simulink subsystem "VCM_main"  (R2021b)
settings: Solver=VariableStepAuto  StartTime=0.0  StopTime=10.0  RelTol=1e-3
undefined symbols (not defined in the file): df, dr, g, gear_f, gear_r, Iwf, Iwr, l, lf, M, Rwf, Rwr
libraries: simulink x47, dspstat3 x2, dspswit3 x1
(part 2 of 4)

== system VCM_main/Sequence/bInberterOn_SwBox1 ==
  BUS : Inport
  error sig1 : Inport  Port=2
  error sig2 : Inport  Port=3
  error sig3 : Inport  Port=4
  error sig4 : Inport  Port=5
  Bus Selector2 : BusSelector  OutputSignals=MC1_sw,MC2_sw,MC3_sw,MC4_sw
  Constant : Constant
  Switch{1..4} (4 alike) : Switch  Criteria=u2 > Threshold
  Out1 : Outport  VectorParamsAs1DForOutWhenUnconnected=off
  Out2 : Outport  Port=2  VectorParamsAs1DForOutWhenUnconnected=off
  Out3 : Outport  Port=3  VectorParamsAs1DForOutWhenUnconnected=off
  Out4 : Outport  Port=4  VectorParamsAs1DForOutWhenUnconnected=off
  wires:
  error sig2/1 -> Switch2/1
  error sig3/1 -> Switch3/1
  error sig4/1 -> Switch4/1
  BUS/1 -> Bus Selector2/1
  Bus Selector2/4 -> Switch4/2  "<MC4_sw>"
  Bus Selector2/3 -> Switch3/2  "<MC3_sw>"
  Bus Selector2/1 -> Switch1/2  "<MC1_sw>"
  Bus Selector2/2 -> Switch2/2  "<MC2_sw>"
  Switch3/1 -> Out3/1
  Switch2/1 -> Out2/1
  error sig1/1 -> Switch1/1
  Switch1/1 -> Out1/1
  Switch4/1 -> Out4/1
  Constant/1 -> Switch1/3, Switch2/3, Switch3/3, Switch4/3

== system VCM_main/Sequence/bQuitDcOn_SwBox ==
  BUS : Inport
  error sig1 : Inport  Port=2
  error sig2 : Inport  Port=3
  error sig3 : Inport  Port=4
  error sig4 : Inport  Port=5
  Bus Selector2 : BusSelector  OutputSignals=MC1_sw,MC2_sw,MC3_sw,MC4_sw
  Constant : Constant
  Switch{1..4} (4 alike) : Switch  Criteria=u2 > Threshold
  Out1 : Outport  VectorParamsAs1DForOutWhenUnconnected=off
  Out2 : Outport  Port=2  VectorParamsAs1DForOutWhenUnconnected=off
  Out3 : Outport  Port=3  VectorParamsAs1DForOutWhenUnconnected=off
  Out4 : Outport  Port=4  VectorParamsAs1DForOutWhenUnconnected=off
  wires:
  error sig2/1 -> Switch2/1
  error sig3/1 -> Switch3/1
  error sig4/1 -> Switch4/1
  BUS/1 -> Bus Selector2/1
  Bus Selector2/4 -> Switch4/2  "<MC4_sw>"
  Bus Selector2/3 -> Switch3/2  "<MC3_sw>"
  Bus Selector2/1 -> Switch1/2  "<MC1_sw>"
  Bus Selector2/2 -> Switch2/2  "<MC2_sw>"
  Switch3/1 -> Out3/1
  Switch2/1 -> Out2/1
  error sig1/1 -> Switch1/1
  Switch1/1 -> Out1/1
  Switch4/1 -> Out4/1
  Constant/1 -> Switch1/3, Switch2/3, Switch3/3, Switch4/3

== system VCM_main/Sequence/bSystemReady_SwBox ==
  BUS : Inport
  error sig1 : Inport  Port=2
  error sig2 : Inport  Port=3
  error sig3 : Inport  Port=4
  error sig4 : Inport  Port=5
  Bus Selector2 : BusSelector  OutputSignals=MC1_sw,MC2_sw,MC3_sw,MC4_sw
  Constant : Constant
  Switch{1..4} (4 alike) : Switch  Criteria=u2 > Threshold
  Out1 : Outport  VectorParamsAs1DForOutWhenUnconnected=off
  Out2 : Outport  Port=2  VectorParamsAs1DForOutWhenUnconnected=off
  Out3 : Outport  Port=3  VectorParamsAs1DForOutWhenUnconnected=off
  Out4 : Outport  Port=4  VectorParamsAs1DForOutWhenUnconnected=off
  wires:
  error sig2/1 -> Switch2/1
  error sig3/1 -> Switch3/1
  error sig4/1 -> Switch4/1
  BUS/1 -> Bus Selector2/1
  Bus Selector2/4 -> Switch4/2  "<MC4_sw>"
  Bus Selector2/3 -> Switch3/2  "<MC3_sw>"
  Bus Selector2/1 -> Switch1/2  "<MC1_sw>"
  Bus Selector2/2 -> Switch2/2  "<MC2_sw>"
  Switch3/1 -> Out3/1
  Switch2/1 -> Out2/1
  error sig1/1 -> Switch1/1
  Switch1/1 -> Out1/1
  Switch4/1 -> Out4/1
  Constant/1 -> Switch1/3, Switch2/3, Switch3/3, Switch4/3

== system VCM_main/Speed Torque MC1/Power limit Negative ==
  Speed : Inport
  Trq : Inport  Port=2
  Constant : Constant  Value=-10000
  Fcn : Fcn  Expr=u(1)/(2*pi*u(2)/60)
  Saturation : Saturate  UpperLimit=30000  LowerLimit=1
  Saturation Dynamic : simulink/Discontinuities/Saturation Dynamic  OutMin=[]  OutMax=[]  OutDataTypeStr=Inherit: Same as second input  OutDataType=fixdt(1, 16)  OutScaling=2^-10  DoSatur=off
  Vector Concatenate : Concatenate
  power limit : Constant  Value=0
  Out1 : Outport  VectorParamsAs1DForOutWhenUnconnected=off
  wires:
  Saturation/1 -> Vector Concatenate/2
  Fcn/1 -> Saturation Dynamic/3
  Vector Concatenate/1 -> Fcn/1
  Constant/1 -> Vector Concatenate/1
  Speed/1 -> Saturation/1
  Saturation Dynamic/1 -> Out1/1
  power limit/1 -> Saturation Dynamic/1
  Trq/1 -> Saturation Dynamic/2

== system VCM_main/Speed Torque MC1/Power limit Positive ==
  note: 80kWPowerLimitがoffのとき
      | モーター1つあたりの出力＊効率
  note: 80kWPowerLimitがonのとき
      | モーター単体最高出力＊効率
  note: PositiveTrqLimitは
      | 単体出力を超えない
      | かつ0以上
  note: 0割り防ぐためだけ
  Trq : Inport
  Speed : Inport  Port=2
  Constant1 : Constant  Value=0
  Fcn : Fcn  Expr=u(1)/(2*pi*u(2)/60)
  Saturation : Saturate  UpperLimit=30000  LowerLimit=1
  Saturation Dynamic : simulink/Discontinuities/Saturation Dynamic  OutMin=[]  OutMax=[]  OutDataTypeStr=Inherit: Same as second input  OutDataType=fixdt(1, 16)  OutScaling=2^-10  DoSatur=off
  Switch : Switch  Criteria=u2 > Threshold  Threshold=0.5
  Vector Concatenate : Concatenate
  all power limit : Constant  Value=35000*0.6
  "each power limit " : Constant  Value=80000/4*0.7
  Out1 : Outport  VectorParamsAs1DForOutWhenUnconnected=off
  wires:
  all power limit/1 -> Switch/1
  "each power limit "/1 -> Switch/3
  [PowerLimitOn] -> Switch/2
  Saturation/1 -> Vector Concatenate/2
  Trq/1 -> Saturation Dynamic/2
  Vector Concatenate/1 -> Fcn/1
  Fcn/1 -> Saturation Dynamic/1
  Switch/1 -> Vector Concatenate/1
  Speed/1 -> Saturation/1
  Saturation Dynamic/1 -> Out1/1
  Constant1/1 -> Saturation Dynamic/3

== system VCM_main/Speed Torque MC1/Subsystem ==
  note: 整数にするときに四捨五入してしまったので
      | インバーターに送って良い最大トルク指令値(0.1%Mn)の2142を
      | 超えることがあるのでminを入れた。
      | 2142より大きい値を送るとエラー出る。
  Positive torque limit : Inport
  M set point MAX 0.1%Mn : Constant  Value=2142
  MinMax : MinMax  Inputs=2
  Positive torque limit1 : Outport  VectorParamsAs1DForOutWhenUnconnected=off
  wires:
  MinMax/1 -> Positive torque limit1/1  "Positive torque limit"
  Positive torque limit/1 -> MinMax/1
  M set point MAX 0.1%Mn/1 -> MinMax/2

== system VCM_main/Speed Torque MC1/TargetVelocity ==
  note: なぜあるかわからん
      | byそが
  note: トルク指令値が正なら
      | SpeedSetpointはTargetSpeedに
      | トルク指令値が負なら
      | SpeedSetpointは0に
  trq : Inport
  target speed : Inport  Port=2
  Constant1 : Constant  Value=0
  Delay : Delay  DelayLength=1  InitialCondition=0
  MinMax : MinMax  Inputs=2
  Switch : Switch  Criteria=u2 > Threshold
  SpeedSetpoint : Outport  VectorParamsAs1DForOutWhenUnconnected=off
  wires:
  MinMax/1 -> SpeedSetpoint/1
  Delay/1 -> MinMax/2
  Switch/1 -> Delay/1, MinMax/1
  Constant1/1 -> Switch/3
  target speed/1 -> Switch/1
  trq/1 -> Switch/2

== system VCM_main/Speed Torque MC1/Torque delay N ==
  In1 : Inport
  Delay : Delay  DelayLength=1  InitialCondition=0
  MinMax : MinMax  Inputs=2
  Out1 : Outport  VectorParamsAs1DForOutWhenUnconnected=off
  wires:
  MinMax/1 -> Out1/1
  Delay/1 -> MinMax/2
  In1/1 -> Delay/1, MinMax/1

== system VCM_main/Speed Torque MC1/Torque delay P ==
  note: なぜあるかわからん
      | byそが
  In1 : Inport
  Delay : Delay  DelayLength=1  InitialCondition=0
  MinMax : MinMax  Function=max  Inputs=2
  Out1 : Outport  VectorParamsAs1DForOutWhenUnconnected=off
  wires:
  MinMax/1 -> Out1/1
  Delay/1 -> MinMax/2
  In1/1 -> Delay/1, MinMax/1

== system VCM_main/Speed Torque MC2/Power limit Negative ==
  Speed : Inport
  Trq : Inport  Port=2
  Constant : Constant  Value=-10000
  Fcn : Fcn  Expr=u(1)/(2*pi*u(2)/60)
  Saturation : Saturate  UpperLimit=30000  LowerLimit=1
  Saturation Dynamic : simulink/Discontinuities/Saturation Dynamic  OutMin=[]  OutMax=[]  OutDataTypeStr=Inherit: Same as second input  OutDataType=fixdt(1, 16)  OutScaling=2^-10  DoSatur=off
  Vector Concatenate : Concatenate
  power limit : Constant  Value=0
  Out1 : Outport  VectorParamsAs1DForOutWhenUnconnected=off
  wires:
  Trq/1 -> Saturation Dynamic/2
  power limit/1 -> Saturation Dynamic/1
  Saturation Dynamic/1 -> Out1/1
  Speed/1 -> Saturation/1
  Constant/1 -> Vector Concatenate/1
  Vector Concatenate/1 -> Fcn/1
  Fcn/1 -> Saturation Dynamic/3
  Saturation/1 -> Vector Concatenate/2

== system VCM_main/Speed Torque MC2/Power limit Positive ==
  note: 0割り防ぐためだけ
  note: PositiveTrqLimitは
      | 単体出力を超えない
      | かつ0以上
  note: 80kWPowerLimitがonのとき
      | モーター単体最高出力＊効率
  note: 80kWPowerLimitがoffのとき
      | モーター1つあたりの出力＊効率
  Trq : Inport
  Speed : Inport  Port=2
  Constant1 : Constant  Value=0
  Fcn : Fcn  Expr=u(1)/(2*pi*u(2)/60)
  Saturation : Saturate  UpperLimit=30000  LowerLimit=1
  Saturation Dynamic : simulink/Discontinuities/Saturation Dynamic  OutMin=[]  OutMax=[]  OutDataTypeStr=Inherit: Same as second input  OutDataType=fixdt(1, 16)  OutScaling=2^-10  DoSatur=off
  Switch : Switch  Criteria=u2 > Threshold  Threshold=0.5
  Vector Concatenate : Concatenate
  all power limit : Constant  Value=35000*0.6
  "each power limit " : Constant  Value=80000/4*0.7
  Out1 : Outport  VectorParamsAs1DForOutWhenUnconnected=off
  wires:
  Constant1/1 -> Saturation Dynamic/3
  Saturation Dynamic/1 -> Out1/1
  Speed/1 -> Saturation/1
  Switch/1 -> Vector Concatenate/1
  Fcn/1 -> Saturation Dynamic/1
  Vector Concatenate/1 -> Fcn/1
  Trq/1 -> Saturation Dynamic/2
  Saturation/1 -> Vector Concatenate/2
  [PowerLimitOn] -> Switch/2
  "each power limit "/1 -> Switch/3
  all power limit/1 -> Switch/1

== system VCM_main/Speed Torque MC2/Subsystem ==
  note: 整数にするときに四捨五入してしまったので
      | インバーターに送って良い最大トルク指令値(0.1%Mn)の2142を
      | 超えることがあるのでminを入れた。
      | 2142より大きい値を送るとエラー出る。
  Positive torque limit : Inport
  M set point MAX 0.1%Mn : Constant  Value=2142
  MinMax : MinMax  Inputs=2
  Positive torque limit1 : Outport  VectorParamsAs1DForOutWhenUnconnected=off
  wires:
  M set point MAX 0.1%Mn/1 -> MinMax/2
  Positive torque limit/1 -> MinMax/1
  MinMax/1 -> Positive torque limit1/1  "Positive torque limit"

== system VCM_main/Speed Torque MC2/TargetVelocity ==
  note: トルク指令値が正なら
      | SpeedSetpointはTargetSpeedに
      | トルク指令値が負なら
      | SpeedSetpointは0に
  note: なぜあるかわからん
      | byそが
  trq : Inport
  target speed : Inport  Port=2
  Constant1 : Constant  Value=0
  Delay : Delay  DelayLength=1  InitialCondition=0
  MinMax : MinMax  Inputs=2
  Switch : Switch  Criteria=u2 > Threshold
  SpeedSetpoint : Outport  VectorParamsAs1DForOutWhenUnconnected=off
  wires:
  trq/1 -> Switch/2
  target speed/1 -> Switch/1
  Constant1/1 -> Switch/3
  Switch/1 -> MinMax/1, Delay/1
  Delay/1 -> MinMax/2
  MinMax/1 -> SpeedSetpoint/1

== system VCM_main/Speed Torque MC2/Torque delay N ==
  In1 : Inport
  Delay : Delay  DelayLength=1  InitialCondition=0
  MinMax : MinMax  Inputs=2
  Out1 : Outport  VectorParamsAs1DForOutWhenUnconnected=off
  wires:
  In1/1 -> MinMax/1, Delay/1
  Delay/1 -> MinMax/2
  MinMax/1 -> Out1/1

== system VCM_main/Speed Torque MC2/Torque delay P ==
  note: なぜあるかわからん
      | byそが
  In1 : Inport
  Delay : Delay  DelayLength=1  InitialCondition=0
  MinMax : MinMax  Function=max  Inputs=2
  Out1 : Outport  VectorParamsAs1DForOutWhenUnconnected=off
  wires:
  In1/1 -> MinMax/1, Delay/1
  Delay/1 -> MinMax/2
  MinMax/1 -> Out1/1

== system VCM_main/Speed Torque MC3/Power limit Negative ==
  Speed : Inport
  Trq : Inport  Port=2
  Constant : Constant  Value=-10000
  Fcn : Fcn  Expr=u(1)/(2*pi*u(2)/60)
  Saturation : Saturate  UpperLimit=30000  LowerLimit=1
  Saturation Dynamic : simulink/Discontinuities/Saturation Dynamic  OutMin=[]  OutMax=[]  OutDataTypeStr=Inherit: Same as second input  OutDataType=fixdt(1, 16)  OutScaling=2^-10  DoSatur=off
  Vector Concatenate : Concatenate
  power limit : Constant  Value=0
  Out1 : Outport  VectorParamsAs1DForOutWhenUnconnected=off
  wires:
  Saturation/1 -> Vector Concatenate/2
  Fcn/1 -> Saturation Dynamic/3
  Vector Concatenate/1 -> Fcn/1
  Constant/1 -> Vector Concatenate/1
  Speed/1 -> Saturation/1
  Saturation Dynamic/1 -> Out1/1
  power limit/1 -> Saturation Dynamic/1
  Trq/1 -> Saturation Dynamic/2

== system VCM_main/Speed Torque MC3/Power limit Positive ==
  note: 80kWPowerLimitがoffのとき
      | モーター1つあたりの出力＊効率
  note: 80kWPowerLimitがonのとき
      | モーター単体最高出力＊効率
  note: PositiveTrqLimitは
      | 単体出力を超えない
      | かつ0以上
  note: 0割り防ぐためだけ
  Trq : Inport
  Speed : Inport  Port=2
  Constant1 : Constant  Value=0
  Fcn : Fcn  Expr=u(1)/(2*pi*u(2)/60)
  Saturation : Saturate  UpperLimit=30000  LowerLimit=1
  Saturation Dynamic : simulink/Discontinuities/Saturation Dynamic  OutMin=[]  OutMax=[]  OutDataTypeStr=Inherit: Same as second input  OutDataType=fixdt(1, 16)  OutScaling=2^-10  DoSatur=off
  Switch : Switch  Criteria=u2 > Threshold  Threshold=0.5
  Vector Concatenate : Concatenate
  all power limit : Constant  Value=35000*0.6
  "each power limit " : Constant  Value=80000/4*0.7
  Out1 : Outport  VectorParamsAs1DForOutWhenUnconnected=off
  wires:
  all power limit/1 -> Switch/1
  "each power limit "/1 -> Switch/3
  [PowerLimitOn] -> Switch/2
  Saturation/1 -> Vector Concatenate/2
  Trq/1 -> Saturation Dynamic/2
  Vector Concatenate/1 -> Fcn/1
  Fcn/1 -> Saturation Dynamic/1
  Switch/1 -> Vector Concatenate/1
  Speed/1 -> Saturation/1
  Saturation Dynamic/1 -> Out1/1
  Constant1/1 -> Saturation Dynamic/3

== system VCM_main/Speed Torque MC3/Subsystem ==
  note: 整数にするときに四捨五入してしまったので
      | インバーターに送って良い最大トルク指令値(0.1%Mn)の2142を
      | 超えることがあるのでminを入れた。
      | 2142より大きい値を送るとエラー出る。
  Positive torque limit : Inport
  M set point MAX 0.1%Mn : Constant  Value=2142
  MinMax : MinMax  Inputs=2
  Positive torque limit1 : Outport  VectorParamsAs1DForOutWhenUnconnected=off
  wires:
  MinMax/1 -> Positive torque limit1/1  "Positive torque limit"
  Positive torque limit/1 -> MinMax/1
  M set point MAX 0.1%Mn/1 -> MinMax/2

== system VCM_main/Speed Torque MC3/TargetVelocity ==
  note: なぜあるかわからん
      | byそが
  note: トルク指令値が正なら
      | SpeedSetpointはTargetSpeedに
      | トルク指令値が負なら
      | SpeedSetpointは0に
  trq : Inport
  target speed : Inport  Port=2
  Constant1 : Constant  Value=0
  Delay : Delay  DelayLength=1  InitialCondition=0
  MinMax : MinMax  Inputs=2
  Switch : Switch  Criteria=u2 > Threshold
  SpeedSetpoint : Outport  VectorParamsAs1DForOutWhenUnconnected=off
  wires:
  MinMax/1 -> SpeedSetpoint/1
  Delay/1 -> MinMax/2
  Switch/1 -> Delay/1, MinMax/1
  Constant1/1 -> Switch/3
  target speed/1 -> Switch/1
  trq/1 -> Switch/2

== system VCM_main/Speed Torque MC3/Torque delay N ==
  In1 : Inport
  Delay : Delay  DelayLength=1  InitialCondition=0
  MinMax : MinMax  Inputs=2
  Out1 : Outport  VectorParamsAs1DForOutWhenUnconnected=off
  wires:
  MinMax/1 -> Out1/1
  Delay/1 -> MinMax/2
  In1/1 -> Delay/1, MinMax/1

== system VCM_main/Speed Torque MC3/Torque delay P ==
  note: なぜあるかわからん
      | byそが
  In1 : Inport
  Delay : Delay  DelayLength=1  InitialCondition=0
  MinMax : MinMax  Function=max  Inputs=2
  Out1 : Outport  VectorParamsAs1DForOutWhenUnconnected=off
  wires:
  MinMax/1 -> Out1/1
  Delay/1 -> MinMax/2
  In1/1 -> Delay/1, MinMax/1

== system VCM_main/Speed Torque MC4/Power limit Negative ==
  Speed : Inport
  Trq : Inport  Port=2
  Constant : Constant  Value=-10000
  Fcn : Fcn  Expr=u(1)/(2*pi*u(2)/60)
  Saturation : Saturate  UpperLimit=30000  LowerLimit=1
  Saturation Dynamic : simulink/Discontinuities/Saturation Dynamic  OutMin=[]  OutMax=[]  OutDataTypeStr=Inherit: Same as second input  OutDataType=fixdt(1, 16)  OutScaling=2^-10  DoSatur=off
  Vector Concatenate : Concatenate
  power limit : Constant  Value=0
  Out1 : Outport  VectorParamsAs1DForOutWhenUnconnected=off
  wires:
  Trq/1 -> Saturation Dynamic/2
  power limit/1 -> Saturation Dynamic/1
  Saturation Dynamic/1 -> Out1/1
  Speed/1 -> Saturation/1
  Constant/1 -> Vector Concatenate/1
  Vector Concatenate/1 -> Fcn/1
  Fcn/1 -> Saturation Dynamic/3
  Saturation/1 -> Vector Concatenate/2

== system VCM_main/Speed Torque MC4/Power limit Positive ==
  note: 0割り防ぐためだけ
  note: PositiveTrqLimitは
      | 単体出力を超えない
      | かつ0以上
  note: 80kWPowerLimitがonのとき
      | モーター単体最高出力＊効率
  note: 80kWPowerLimitがoffのとき
      | モーター1つあたりの出力＊効率
  Trq : Inport
  Speed : Inport  Port=2
  Constant1 : Constant  Value=0
  Fcn : Fcn  Expr=u(1)/(2*pi*u(2)/60)
  Saturation : Saturate  UpperLimit=30000  LowerLimit=1
  Saturation Dynamic : simulink/Discontinuities/Saturation Dynamic  OutMin=[]  OutMax=[]  OutDataTypeStr=Inherit: Same as second input  OutDataType=fixdt(1, 16)  OutScaling=2^-10  DoSatur=off
  Switch : Switch  Criteria=u2 > Threshold  Threshold=0.5
  Vector Concatenate : Concatenate
  all power limit : Constant  Value=35000*0.6
  "each power limit " : Constant  Value=80000/4*0.7
  Out1 : Outport  VectorParamsAs1DForOutWhenUnconnected=off
  wires:
  Constant1/1 -> Saturation Dynamic/3
  Saturation Dynamic/1 -> Out1/1
  Speed/1 -> Saturation/1
  Switch/1 -> Vector Concatenate/1
  Fcn/1 -> Saturation Dynamic/1
  Vector Concatenate/1 -> Fcn/1
  Trq/1 -> Saturation Dynamic/2
  Saturation/1 -> Vector Concatenate/2
  [PowerLimitOn] -> Switch/2
  "each power limit "/1 -> Switch/3
  all power limit/1 -> Switch/1

== system VCM_main/Speed Torque MC4/Subsystem ==
  note: 整数にするときに四捨五入してしまったので
      | インバーターに送って良い最大トルク指令値(0.1%Mn)の2142を
      | 超えることがあるのでminを入れた。
      | 2142より大きい値を送るとエラー出る。
  Positive torque limit : Inport
  M set point MAX 0.1%Mn : Constant  Value=2142
  MinMax : MinMax  Inputs=2
  Positive torque limit1 : Outport  VectorParamsAs1DForOutWhenUnconnected=off
  wires:
  M set point MAX 0.1%Mn/1 -> MinMax/2
  Positive torque limit/1 -> MinMax/1
  MinMax/1 -> Positive torque limit1/1  "Positive torque limit"

== system VCM_main/Speed Torque MC4/TargetVelocity ==
  note: トルク指令値が正なら
      | SpeedSetpointはTargetSpeedに
      | トルク指令値が負なら
      | SpeedSetpointは0に
  note: なぜあるかわからん
      | byそが
  trq : Inport
  target speed : Inport  Port=2
  Constant1 : Constant  Value=0
  Delay : Delay  DelayLength=1  InitialCondition=0
  MinMax : MinMax  Inputs=2
  Switch : Switch  Criteria=u2 > Threshold
  SpeedSetpoint : Outport  VectorParamsAs1DForOutWhenUnconnected=off
  wires:
  trq/1 -> Switch/2
  target speed/1 -> Switch/1
  Constant1/1 -> Switch/3
  Switch/1 -> MinMax/1, Delay/1
  Delay/1 -> MinMax/2
  MinMax/1 -> SpeedSetpoint/1

== system VCM_main/Speed Torque MC4/Torque delay N ==
  In1 : Inport
  Delay : Delay  DelayLength=1  InitialCondition=0
  MinMax : MinMax  Inputs=2
  Out1 : Outport  VectorParamsAs1DForOutWhenUnconnected=off
  wires:
  In1/1 -> MinMax/1, Delay/1
  Delay/1 -> MinMax/2
  MinMax/1 -> Out1/1

== system VCM_main/Speed Torque MC4/Torque delay P ==
  note: なぜあるかわからん
      | byそが
  In1 : Inport
  Delay : Delay  DelayLength=1  InitialCondition=0
  MinMax : MinMax  Function=max  Inputs=2
  Out1 : Outport  VectorParamsAs1DForOutWhenUnconnected=off
  wires:
  In1/1 -> MinMax/1, Delay/1
  Delay/1 -> MinMax/2
  MinMax/1 -> Out1/1

== system VCM_main/VDC/80kw_limitation ==
  TrqIn : Inport
  Power Consumption : Inport  Port=2
  Eff_INV : Gain  Gain=98/100
  Max Power : Constant  Value=70000
  Power Limit{,1..4} (5 alike) : Subsystem  ReferencedSubsystem=Power_Limit
  Power Limit_last : Subsystem
  Scope : Scope  NumInputPorts=5
  signal select : Subsystem
  TrqOut : Outport  VectorParamsAs1DForOutWhenUnconnected=off
  wires:
  Power Limit_last/1(TrqOut) -> TrqOut/1
  Power Limit4/2 -> Scope/5
  Power Limit3/2 -> Scope/4
  Power Limit2/2 -> Scope/3
  Power Limit1/2 -> Scope/2
  Power Limit/2 -> Scope/1
  Eff_INV/1 -> Power Limit3/2, Power Limit4/2, Power Limit2/2, Power Limit1/2, Power Limit/2
  Max Power/1 -> Eff_INV/1
  Power Limit4/1 -> Power Limit_last/1(LimitTorque)
  Power Limit3/1 -> Power Limit4/1
  Power Limit2/1 -> Power Limit3/1
  Power Limit1/1 -> Power Limit2/1
  Power Limit/1 -> Power Limit1/1
  Power Consumption/1 -> Power Limit_last/2(Power Consumption)
  TrqIn/1 -> Power Limit_last/3(Torque), signal select/1(Torque)
  signal select/1(Torque Speed) -> Power Limit/1

== system VCM_main/VDC/DYC1 ==
  Total Torque In : Inport
  DriverInput : Inport  Port=2
  Sensor : Inport  Port=3
  Bus Creator : BusCreator  Inputs=2
  Bus Selector : BusSelector  OutputSignals=TrqOut_f,TrqOut_r
  DYC Switch : Subsystem
  DYC Switch1 : Subsystem
  DYC Switch2 : Subsystem
  DYC Switch3 : Subsystem
  DYC Torque : Scope  NumInputPorts=4
  DYC main : Subsystem
  DYC_Output : Outport
  RRtorque : Outport  Port=2
  RLtorque : Outport  Port=3
  FRtorque : Outport  Port=4
  FLtorque : Outport  Port=5
  wires:
  DYC main/4(DYC_FL) -> DYC Switch3/2(DYC_Torque)
  DYC main/3(DYC_FR) -> DYC Switch2/2(DYC_Torque)
  DYC main/2(DYC_RL) -> DYC Switch1/2(DYC_Torque)
  DYC main/1(DYC_RR) -> DYC Switch/2(DYC_Torque)
  DYC main/6(Moment) -> Bus Creator/2
  DYC main/5(Gain) -> Bus Creator/1
  Sensor/1 -> DYC main/3(Sensor)
  DriverInput/1 -> DYC main/2(DriverInput)
  Bus Selector/1 -> DYC Switch1/1(Torque In), DYC Switch/1(Torque In)  "<TrqOut_f>"
  Total Torque In/1 -> DYC main/1(Total Torque In), Bus Selector/1  "Total Torque In"
  Bus Selector/2 -> DYC Switch2/1(Torque In), DYC Switch3/1(Torque In)  "<TrqOut_r>"
  Bus Creator/1 -> DYC_Output/1  "DYC_Output"
  DYC Switch2/1(torque) -> FRtorque/1, DYC Torque/3  "FRtorque"
  DYC Switch1/1(torque) -> RLtorque/1, DYC Torque/2  "RLtorque"
  DYC Switch/1(torque) -> RRtorque/1, DYC Torque/1  "RRtorque"
  DYC Switch3/1(torque) -> FLtorque/1, DYC Torque/4  "FLtorque"

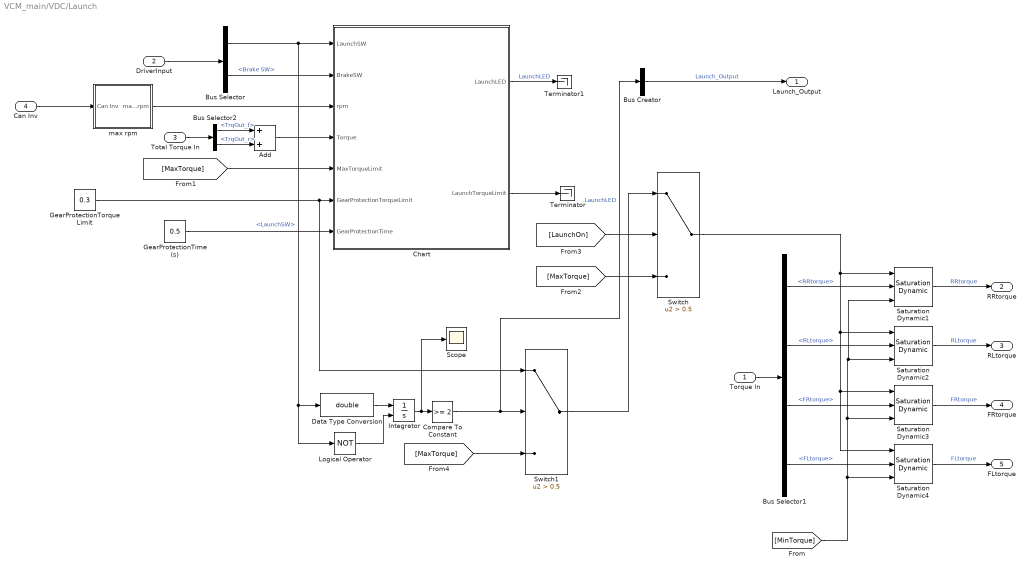
== system VCM_main/VDC/Launch ==
  Torque In : Inport
  DriverInput : Inport  Port=2
  Total Torque In : Inport  Port=3
  Can Inv : Inport  Port=4
  Add : Sum
  Bus Creator : BusCreator  Inputs=1
  Bus Selector : BusSelector  OutputSignals=LaunchSW,Brake SW
  Bus Selector1 : BusSelector  OutputSignals=RRtorque,RLtorque,FRtorque,FLtorque
  Bus Selector2 : BusSelector  OutputSignals=TrqOut_f,TrqOut_r
  Chart : Stateflow chart  TreatAsAtomicUnit=on
  Compare To Constant : simulink/Logic and Bit Operations/Compare To Constant  relop=>=  const=2  OutDataTypeStr=boolean
  Data Type Conversion : DataTypeConversion  OutDataTypeStr=double
  GearProtectionTime (s) : Constant  Value=0.5
  GearProtectionTorqueLimit : Constant  Value=0.3
  Integrator : Integrator  ExternalReset=rising
  Logical Operator : Logic  Operator=NOT  AllPortsSameDT=off  OutDataTypeStr=boolean
  Saturation Dynamic{1..4} (4 alike) : simulink/Discontinuities/Saturation Dynamic  OutMin=[]  OutMax=[]  OutDataTypeStr=Inherit: Same as second input  OutDataType=fixdt(1, 16)  OutScaling=2^-10  DoSatur=off
  Scope : Scope
  Switch : Switch  Criteria=u2 > Threshold  Threshold=0.5
  Switch1 : Switch  Criteria=u2 > Threshold  Threshold=0.5
  Terminator : Terminator
  Terminator1 : Terminator
  max rpm : Subsystem
  Launch_Output : Outport
  RRtorque : Outport  Port=2
  RLtorque : Outport  Port=3
  FRtorque : Outport  Port=4
  FLtorque : Outport  Port=5
  wires:
  Add/1 -> Chart/4(Torque)
  Bus Selector2/2 -> Add/2  "<TrqOut_r>"
  Bus Selector2/1 -> Add/1  "<TrqOut_f>"
  Data Type Conversion/1 -> Integrator/1
  Switch1/1 -> Switch/1
  Compare To Constant/1 -> Switch1/2, Bus Creator/1  "LaunchLED"
  Logical Operator/1 -> Integrator/2
  GearProtectionTorqueLimit/1 -> Chart/6(GearProtectionTorqueLimit), Switch1/1
  [MaxTorque] -> Switch1/3
  Integrator/1 -> Compare To Constant/1, Scope/1
  [LaunchOn] -> Switch/2
  [MaxTorque] -> Switch/3
  Chart/2(LaunchTorqueLimit) -> Terminator/1
  Chart/1(LaunchLED) -> Terminator1/1  "LaunchLED"
  Bus Creator/1 -> Launch_Output/1  "Launch_Output"
  Total Torque In/1 -> Bus Selector2/1
  max rpm/1(max rpm) -> Chart/3(rpm)
  Can Inv/1 -> max rpm/1(Can Inv)
  Bus Selector/2 -> Chart/2(BrakeSW)  "<Brake SW>"
  Bus Selector/1 -> Chart/1(LaunchSW), Data Type Conversion/1, Logical Operator/1  "<LaunchSW>"
  DriverInput/1 -> Bus Selector/1
  GearProtectionTime (s)/1 -> Chart/7(GearProtectionTime)
  [MaxTorque] -> Chart/5(MaxTorqueLimit)
  [MinTorque] -> Saturation Dynamic4/3, Saturation Dynamic3/3, Saturation Dynamic2/3, Saturation Dynamic1/3
  Switch/1 -> Saturation Dynamic1/1, Saturation Dynamic2/1, Saturation Dynamic3/1, Saturation Dynamic4/1
  Saturation Dynamic1/1 -> RRtorque/1  "RRtorque"
  Torque In/1 -> Bus Selector1/1
  Saturation Dynamic2/1 -> RLtorque/1  "RLtorque"
  Saturation Dynamic3/1 -> FRtorque/1  "FRtorque"
  Saturation Dynamic4/1 -> FLtorque/1  "FLtorque"
  Bus Selector1/3 -> Saturation Dynamic3/2  "<FRtorque>"
  Bus Selector1/1 -> Saturation Dynamic1/2  "<RRtorque>"
  Bus Selector1/2 -> Saturation Dynamic2/2  "<RLtorque>"
  Bus Selector1/4 -> Saturation Dynamic4/2  "<FLtorque>"

== system VCM_main/VDC/PowerConsumption ==
  note: ACC Current
  from INV : Inport
  Sensor : Inport  Port=2
  Bus Selector : BusSelector  OutputSignals=IVT_Msg_Result_I
  Bus Selector1 : BusSelector  OutputSignals=MC_11.MC1_DC bus voltage,MC_21.MC2_DC bus voltage,MC_31.MC3_DC bus voltage,MC_41.MC4_DC bus voltage
  Gain : Gain  Gain=100
  Max : MinMax  Function=max  Inputs=4
  Product : Product
  Out1 : Outport  VectorParamsAs1DForOutWhenUnconnected=off
  wires:
  Bus Selector/1 -> Gain/1  "<IVT_Msg_Result_I>"
  Sensor/1 -> Bus Selector/1
  Max/1 -> Product/1
  Bus Selector1/4 -> Max/4  "<MC4_DC bus voltage>"
  Bus Selector1/3 -> Max/3  "<MC3_DC bus voltage>"
  Bus Selector1/2 -> Max/2  "<MC2_DC bus voltage>"
  Bus Selector1/1 -> Max/1  "<MC1_DC bus voltage>"
  Product/1 -> Out1/1
  from INV/1 -> Bus Selector1/1
  Gain/1 -> Product/2

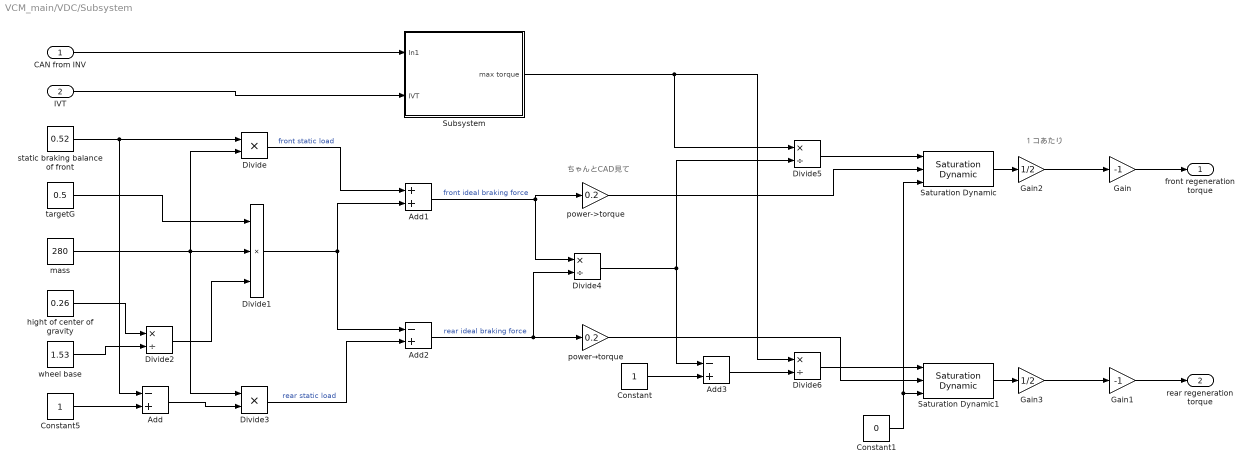
== system VCM_main/VDC/Subsystem ==
  note: ちゃんとCAD見て
  note: １コあたり
  CAN from INV : Inport
  IVT : Inport  Port=2
  Add : Sum  Inputs=-+
  Add1 : Sum
  Add2 : Sum  Inputs=-+
  Add3 : Sum  Inputs=-+
  Constant : Constant
  Constant1 : Constant  Value=0
  Constant5 : Constant
  Divide : Product  Inputs=**
  Divide1 : Product  Inputs=***
  Divide{2,4..6} (4 alike) : Product  Inputs=*/
  Divide3 : Product  Inputs=**
  Gain : Gain  Gain=-1
  Gain1 : Gain  Gain=-1
  Gain2 : Gain  Gain=1/2
  Gain3 : Gain  Gain=1/2
  Saturation Dynamic : simulink/Discontinuities/Saturation Dynamic  OutMin=[]  OutMax=[]  OutDataTypeStr=Inherit: Same as second input  OutDataType=fixdt(1, 16)  OutScaling=2^-10  DoSatur=off
  Saturation Dynamic1 : simulink/Discontinuities/Saturation Dynamic  OutMin=[]  OutMax=[]  OutDataTypeStr=Inherit: Same as second input  OutDataType=fixdt(1, 16)  OutScaling=2^-10  DoSatur=off
  Subsystem : Subsystem
  hight of center of gravity : Constant  Value=0.26
  mass : Constant  Value=280
  power->torque : Gain  Gain=0.2
  power→torque : Gain  Gain=0.2
  static braking balance of front : Constant  Value=0.52
  targetG : Constant  Value=0.5
  wheel base : Constant  Value=1.53
  front regeneration torque : Outport
  rear regeneration torque : Outport  Port=2
  wires:
  Gain3/1 -> Gain1/1
  Gain2/1 -> Gain/1
  power→torque/1 -> Saturation Dynamic1/2
  power->torque/1 -> Saturation Dynamic/2
  Gain1/1 -> rear regeneration torque/1
  Gain/1 -> front regeneration torque/1
  Saturation Dynamic/1 -> Gain2/1
  Saturation Dynamic1/1 -> Gain3/1
  Constant1/1 -> Saturation Dynamic1/3, Saturation Dynamic/3
  Divide6/1 -> Saturation Dynamic1/1
  Divide5/1 -> Saturation Dynamic/1
  Subsystem/1(max torque) -> Divide5/1, Divide6/1
  IVT/1 -> Subsystem/2(IVT)
  CAN from INV/1 -> Subsystem/1(In1)
  Divide4/1 -> Divide5/2, Add3/1
  Add3/1 -> Divide6/2
  Constant/1 -> Add3/2
  Add2/1 -> Divide4/2, power→torque/1  "rear ideal braking force"
  Add1/1 -> Divide4/1, power->torque/1  "front ideal braking force"
  Divide1/1 -> Add2/1, Add1/2
  Divide3/1 -> Add2/2  "rear static load"
  Divide/1 -> Add1/1  "front static load"
  Add/1 -> Divide3/2
  Constant5/1 -> Add/2
  Divide2/1 -> Divide1/3
  wheel base/1 -> Divide2/2
  hight of center of gravity/1 -> Divide2/1
  mass/1 -> Divide1/2, Divide/2, Divide3/1
  targetG/1 -> Divide1/1
  static braking balance of front/1 -> Add/1, Divide/1

== system VCM_main/VDC/Subsystem1 ==
  CAN from INV : Inport
  IVT : Inport  Port=2
  Sensor : Inport  Port=3
  Driver : Inport  Port=4
  Add : Sum  Inputs=+-
  Add1 : Sum  Inputs=+-
  Add3 : Sum  Inputs=-+
  Bus Selector : BusSelector  OutputSignals=BrakePressF,BrakePressR
  Constant : Constant
  Constant1 : Constant  Value=0
  Constant2 : Constant  Value=0
  Divide4 : Product  Inputs=*/
  Divide5 : Product  Inputs=*/
  Divide6 : Product  Inputs=*/
  Gain : Gain  Gain=-1
  Gain1 : Gain  Gain=-1
  Saturation Dynamic : simulink/Discontinuities/Saturation Dynamic  OutMin=[]  OutMax=[]  OutDataTypeStr=Inherit: Same as second input  OutDataType=fixdt(1, 16)  OutScaling=2^-10  DoSatur=off
  Saturation Dynamic1 : simulink/Discontinuities/Saturation Dynamic  OutMin=[]  OutMax=[]  OutDataTypeStr=Inherit: Same as second input  OutDataType=fixdt(1, 16)  OutScaling=2^-10  DoSatur=off
  Subsystem : Subsystem
  Switch : Switch  Criteria=u2 > Threshold
  Switch1 : Switch  Criteria=u2 > Threshold
  ideal brake torque for real time : Subsystem
  front regeneration torque : Outport
  rear regeneration torque : Outport  Port=2
  wires:
  [ReGenerationBrakeOn] -> Switch1/2, Switch/2
  Constant2/1 -> Switch1/3, Switch/3
  Switch/1 -> front regeneration torque/1
  Switch1/1 -> rear regeneration torque/1
  Add/1 -> Saturation Dynamic/2
  Bus Selector/1 -> Add/2  "<BrakePressF>"
  Add1/1 -> Saturation Dynamic1/2
  Bus Selector/2 -> Add1/2  "<BrakePressR>"
  Driver/1 -> Bus Selector/1
  Sensor/1 -> ideal brake torque for real time/1(In1)
  ideal brake torque for real time/2(rear ideal braking torque) -> Add1/1, Divide4/2
  ideal brake torque for real time/1(front ideal braking torque) -> Add/1, Divide4/1
  Gain1/1 -> Switch1/1
  Gain/1 -> Switch/1
  Saturation Dynamic/1 -> Gain/1
  Saturation Dynamic1/1 -> Gain1/1
  Constant1/1 -> Saturation Dynamic1/3, Saturation Dynamic/3
  Divide6/1 -> Saturation Dynamic1/1
  Divide5/1 -> Saturation Dynamic/1
  Subsystem/1(Out1) -> Divide5/1, Divide6/1
  IVT/1 -> Subsystem/2(IVT)
  CAN from INV/1 -> Subsystem/1(CAN from INV)
  Divide4/1 -> Divide5/2, Add3/1
  Add3/1 -> Divide6/2
  Constant/1 -> Add3/2

== system VCM_main/VDC/Subsystem2 ==
  Torque by Accel : Inport
  brake : Inport  Port=2
  Torque by Brake : Inport  Port=3
  Bus Selector : BusSelector  OutputSignals=Brake SW
  Switch : Switch  Criteria=u2 > Threshold
  Total Torque In : Outport
  wires:
  Bus Selector/1 -> Switch/2  "<Brake SW>"
  Switch/1 -> Total Torque In/1
  Torque by Brake/1 -> Switch/3
  Torque by Accel/1 -> Switch/1
  brake/1 -> Bus Selector/1

== system VCM_main/VDC/Torque Front//rear distributor Main ==
  note: FEM20
      | 番号タイヤ対応表
      | 1:FR 2:RR
      | 3:RL 4:FL
  Sensor : Inport
  Total Torque In : Inport  Port=2
  InvSw : Inport  Port=3
  Bus Selector : BusSelector  OutputSignals=MC2_sw,MC3_sw,MC1_sw,MC4_sw
  Bus Selector1 : BusSelector  OutputSignals=CAN_from_IMU_121.ACCEL_X
  Constant : Constant  Value=0
  Max Torque Limit : Subsystem
  Min Torque Limit : Subsystem
  Saturation : Subsystem
  Scope : Scope  NumInputPorts=2
  Switch : Switch  Criteria=u2 > Threshold  Threshold=0.5
  Switch1 : Switch  Criteria=u2 > Threshold  Threshold=0.5
  Switch{2..5} (4 alike) : Switch  Criteria=u2 > Threshold
  "Torque Front/rear distributor " : Subsystem
  Transfer Fcn : TransferFcn  Denominator=[0.03 1]
  Trq F/R Dist Gain : Constant  Value=0.8
  RRtorque : Outport
  RLtorque : Outport  Port=2
  FRtorque : Outport  Port=3
  FLtorque : Outport  Port=4
  wires:
  Bus Selector/4 -> Switch5/2  "<MC4_sw>"
  Bus Selector/3 -> Switch4/2  "<MC1_sw>"
  Bus Selector/2 -> Switch3/2  "<MC3_sw>"
  Constant/1 -> Switch2/3, Switch3/3, Switch4/3, Switch5/3
  Bus Selector/1 -> Switch2/2  "<MC2_sw>"
  InvSw/1 -> Bus Selector/1
  Total Torque In/1 -> Saturation/1(u)
  Saturation/1(y) -> Switch/3, Switch1/3, "Torque Front/rear distributor "/2(Total Torque In)
  [MinTorque] -> Min Torque Limit/1(Min Torque)
  [MaxTorque] -> Max Torque Limit/1(Max Torque)
  Switch3/1 -> RLtorque/1  "RLtorque"
  "Torque Front/rear distributor "/2(torque_rear) -> Max Torque Limit/3(torque_rear)
  Switch5/1 -> FLtorque/1  "FLtorque"
  Max Torque Limit/1(torque_front Out) -> Min Torque Limit/2(torque_front)
  Switch4/1 -> FRtorque/1  "FRtorque"
  Switch1/1 -> Switch2/1, Switch3/1
  Min Torque Limit/2(torque_front Out) -> Scope/2, Switch/1  "torque_front"
  Bus Selector1/1 -> Transfer Fcn/1  "<ACCEL_X>"
  "Torque Front/rear distributor "/1(torque_front) -> Max Torque Limit/2(torque_front)
  Switch2/1 -> RRtorque/1  "RRtorque"
  Trq F/R Dist Gain/1 -> "Torque Front/rear distributor "/3(Trq F/R Dist Gain)
  Min Torque Limit/1(torque_rear Out) -> Scope/1, Switch1/1  "torque_rear"
  Sensor/1 -> Bus Selector1/1
  [F_RTrqDistOn] -> Switch/2, Switch1/2
  Transfer Fcn/1 -> "Torque Front/rear distributor "/1(ACCEL_X)
  Max Torque Limit/2(torque_rear Out) -> Min Torque Limit/3(torque_rear)
  Switch/1 -> Switch4/1, Switch5/1

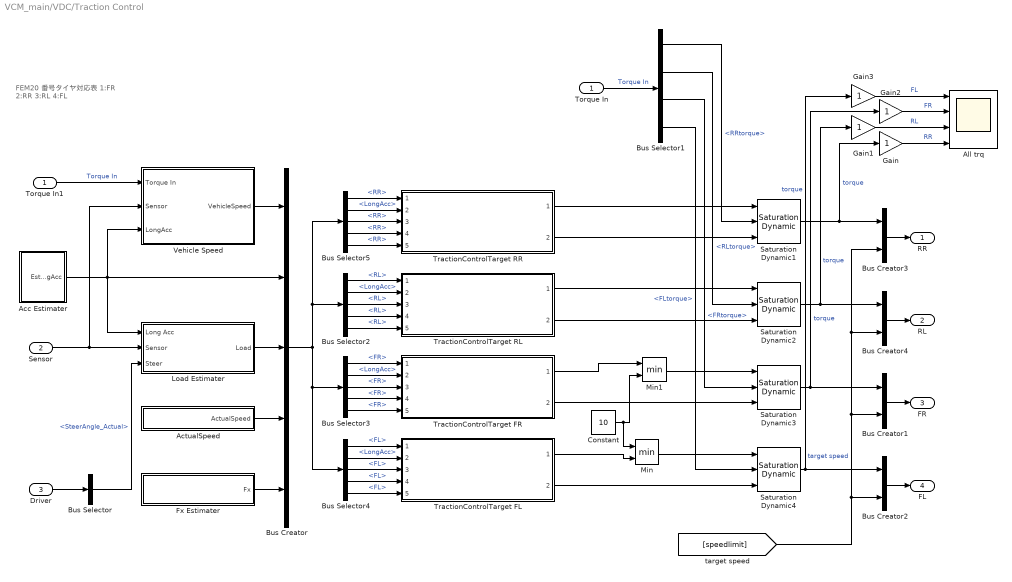
== system VCM_main/VDC/Traction Control ==
  note: FEM20
      | 番号タイヤ対応表
      | 1:FR 2:RR
      | 3:RL 4:FL
  Torque In : Inport
  Sensor : Inport  Port=2
  Driver : Inport  Port=3
  Acc Estimater : Subsystem
  ActualSpeed : Subsystem
  All trq : Scope  NumInputPorts=4
  Bus Creator : BusCreator  Inputs=5
  Bus Creator{1..4} (4 alike) : BusCreator  Inputs=2
  Bus Selector : BusSelector  OutputSignals=SteerAngle_Actual
  Bus Selector1 : BusSelector  OutputSignals=RRtorque,RLtorque,FRtorque,FLtorque
  Bus Selector2 : BusSelector  OutputSignals=VehicleSpeed.RL,LongAcc,Load.RL,Fx.RL,ActualSpeed.RL
  Bus Selector3 : BusSelector  OutputSignals=VehicleSpeed.FR,LongAcc,Load.FR,Fx.FR,ActualSpeed.FR
  Bus Selector4 : BusSelector  OutputSignals=VehicleSpeed.FL,LongAcc,Load.FL,Fx.FL,ActualSpeed.FL
  Bus Selector5 : BusSelector  OutputSignals=VehicleSpeed.RR,LongAcc,Load.RR,Fx.RR,ActualSpeed.RR
  Constant : Constant  Value=10
  Fx Estimater : Subsystem
  Gain{,1..3} (4 alike) : Gain
  Load Estimater : Subsystem
  Min : MinMax  Inputs=2
  Min1 : MinMax  Inputs=2
  Saturation Dynamic{1..4} (4 alike) : simulink/Discontinuities/Saturation Dynamic  OutMin=[]  OutMax=[]  OutDataTypeStr=Inherit: Same as second input  OutDataType=fixdt(1, 16)  OutScaling=2^-10  DoSatur=off
  Torque In1 : InportShadow
  TractionControlTarget FL : Subsystem  ReferencedSubsystem=TC_Target
  TractionControlTarget FR : Subsystem  ReferencedSubsystem=TC_Target
  TractionControlTarget RL : Subsystem  ReferencedSubsystem=TC_Target
  TractionControlTarget RR : Subsystem  ReferencedSubsystem=TC_Target
  Vehicle Speed : Subsystem
  RR : Outport  VectorParamsAs1DForOutWhenUnconnected=off
  RL : Outport  Port=2  VectorParamsAs1DForOutWhenUnconnected=off
  FR : Outport  Port=3  VectorParamsAs1DForOutWhenUnconnected=off
  FL : Outport  Port=4  VectorParamsAs1DForOutWhenUnconnected=off
  wires:
  Torque In1/1 -> Vehicle Speed/1(Torque In)  "Torque In"
  Vehicle Speed/1(VehicleSpeed) -> Bus Creator/1
  Bus Selector/1 -> Load Estimater/3(Steer)  "<SteerAngle_Actual>"
  Driver/1 -> Bus Selector/1
  Bus Selector4/1 -> TractionControlTarget FL/1  "<FL>"
  Bus Selector3/1 -> TractionControlTarget FR/1  "<FR>"
  Bus Selector2/1 -> TractionControlTarget RL/1  "<RL>"
  Bus Selector5/1 -> TractionControlTarget RR/1  "<RR>"
  Torque In/1 -> Bus Selector1/1  "Torque In"
  Bus Creator3/1 -> RR/1
  [speedlimit] -> Bus Creator4/2, Bus Creator3/2, Bus Creator1/2, Bus Creator2/2  "target speed"
  Min1/1 -> Saturation Dynamic3/1
  Constant/1 -> Min1/2, Min/1
  Min/1 -> Saturation Dynamic4/1
  Acc Estimater/1(EstLongAcc) -> Vehicle Speed/3(LongAcc), Bus Creator/2, Load Estimater/1(Long Acc)
  Gain3/1 -> All trq/1  "FL"
  Gain2/1 -> All trq/2  "FR"
  Gain1/1 -> All trq/3  "RL"
  Gain/1 -> All trq/4  "RR"
  Bus Creator2/1 -> FL/1
  Bus Creator1/1 -> FR/1
  Saturation Dynamic4/1 -> Gain3/1, Bus Creator2/1  "torque"
  Saturation Dynamic3/1 -> Gain2/1, Bus Creator1/1  "torque"
  Bus Creator4/1 -> RL/1
  Saturation Dynamic2/1 -> Bus Creator4/1, Gain1/1  "torque"
  ActualSpeed/1(ActualSpeed) -> Bus Creator/4
  Bus Creator/1 -> Bus Selector5/1, Bus Selector2/1, Bus Selector4/1, Bus Selector3/1
  Bus Selector2/4 -> TractionControlTarget RL/4  "<RL>"
  Bus Selector2/3 -> TractionControlTarget RL/3  "<RL>"
  Bus Selector2/2 -> TractionControlTarget RL/2  "<LongAcc>"
  Bus Selector2/5 -> TractionControlTarget RL/5  "<RL>"
  Bus Selector3/4 -> TractionControlTarget FR/4  "<FR>"
  Bus Selector3/3 -> TractionControlTarget FR/3  "<FR>"
  Bus Selector3/2 -> TractionControlTarget FR/2  "<LongAcc>"
  Bus Selector3/5 -> TractionControlTarget FR/5  "<FR>"
  Bus Selector4/4 -> TractionControlTarget FL/4  "<FL>"
  Bus Selector4/3 -> TractionControlTarget FL/3  "<FL>"
  Bus Selector4/2 -> TractionControlTarget FL/2  "<LongAcc>"
  Bus Selector4/5 -> TractionControlTarget FL/5  "<FL>"
  Bus Selector5/5 -> TractionControlTarget RR/5  "<RR>"
  Bus Selector5/4 -> TractionControlTarget RR/4  "<RR>"
  Bus Selector5/3 -> TractionControlTarget RR/3  "<RR>"
  Bus Selector5/2 -> TractionControlTarget RR/2  "<LongAcc>"
  Bus Selector1/1 -> Saturation Dynamic1/2  "<RRtorque>"
  Bus Selector1/2 -> Saturation Dynamic2/2  "<RLtorque>"
  Bus Selector1/3 -> Saturation Dynamic3/2  "<FRtorque>"
  Bus Selector1/4 -> Saturation Dynamic4/2  "<FLtorque>"
  Fx Estimater/1(Fx) -> Bus Creator/5
  Load Estimater/1(Load) -> Bus Creator/3
  Saturation Dynamic1/1 -> Bus Creator3/1, Gain/1  "torque"
  Sensor/1 -> Vehicle Speed/2(Sensor), Load Estimater/2(Sensor)
  TractionControlTarget FL/1 -> Min/2
  TractionControlTarget FL/2 -> Saturation Dynamic4/3
  TractionControlTarget FR/1 -> Min1/1
  TractionControlTarget FR/2 -> Saturation Dynamic3/3
  TractionControlTarget RL/1 -> Saturation Dynamic2/1
  TractionControlTarget RL/2 -> Saturation Dynamic2/3
  TractionControlTarget RR/2 -> Saturation Dynamic1/3
  TractionControlTarget RR/1 -> Saturation Dynamic1/1

== system VCM_main/VDC/VCM_Status ==
  <VDCSW> : Inport
  Sensor : Inport  Port=2
  DYC_Output : Inport  Port=3
  Launch_Output : Inport  Port=4
  power consumption : Inport  Port=5
  trq_VDC : Inport  Port=6
  Bus Creator2 : BusCreator  Inputs=6
  Bus Selector : BusSelector  Commented=on  OutputSignals=LaunchLED
  Gain : Gain  Gain=0.001
  Sliprate : Subsystem
  Terminator : Terminator
  VCMStatus_bus : Subsystem
  VCMStatus : Outport  VectorParamsAs1DForOutWhenUnconnected=off
  wires:
  Sliprate/1(Sliprate) -> Bus Creator2/6  "Sliprate"
  Sensor/1 -> Sliprate/1(from Sensor)
  Bus Creator2/1 -> VCMStatus/1
  power consumption/1 -> Gain/1  "power consumption"
  trq_VDC/1 -> Bus Creator2/5
  <VDCSW>/1 -> VCMStatus_bus/1(In1)
  Gain/1 -> Bus Creator2/4  "power consumption(kW)"
  DYC_Output/1 -> Bus Creator2/2
  VCMStatus_bus/1(VCMStatus) -> Bus Creator2/1
  Launch_Output/1 -> Bus Selector/1
  Bus Selector/1 -> Terminator/1  "<LaunchLED>"

== system VCM_main/Error display Box/Error Info/error memory MC1 ==
  Error info : Inport
  Compare To Zero : simulink/Logic and Bit Operations/Compare To Zero  relop=~=  OutDataTypeStr=boolean
  Compare To Zero1 : simulink/Logic and Bit Operations/Compare To Zero  relop=~=  OutDataTypeStr=boolean
  Logical Operator : Logic  AllPortsSameDT=off  OutDataTypeStr=boolean
  Memory : Memory
  Sum : Sum  Inputs=|+-
  Triggered Subsystem : Subsystem  TreatAsAtomicUnit=on
  error1 : Outport  VectorParamsAs1DForOutWhenUnconnected=off
  error2 : Outport  Port=2  VectorParamsAs1DForOutWhenUnconnected=off
  error3 : Outport  Port=3  VectorParamsAs1DForOutWhenUnconnected=off
  error triger : Outport  Port=4  VectorParamsAs1DForOutWhenUnconnected=off
  wires:
  Triggered Subsystem/3(Out3) -> error3/1
  Sum/1 -> Compare To Zero/1
  Compare To Zero/1 -> Logical Operator/2
  Triggered Subsystem/2(Out2) -> error2/1
  Compare To Zero1/1 -> Logical Operator/1
  Logical Operator/1 -> Triggered Subsystem/Trigger, error triger/1
  Triggered Subsystem/1(Out1) -> error1/1, Memory/1
  Memory/1 -> Sum/2
  Error info/1 -> Sum/1, Triggered Subsystem/1(In1), Compare To Zero1/1

== system VCM_main/Error display Box/Error Info/error memory MC2 ==
  Error info : Inport
  Compare To Zero : simulink/Logic and Bit Operations/Compare To Zero  relop=~=  OutDataTypeStr=boolean
  Compare To Zero1 : simulink/Logic and Bit Operations/Compare To Zero  relop=~=  OutDataTypeStr=boolean
  Logical Operator : Logic  AllPortsSameDT=off  OutDataTypeStr=boolean
  Memory : Memory
  Sum : Sum  Inputs=|+-
  Triggered Subsystem : Subsystem  TreatAsAtomicUnit=on
  error1 : Outport  VectorParamsAs1DForOutWhenUnconnected=off
  error2 : Outport  Port=2  VectorParamsAs1DForOutWhenUnconnected=off
  error3 : Outport  Port=3  VectorParamsAs1DForOutWhenUnconnected=off
  error triger : Outport  Port=4  VectorParamsAs1DForOutWhenUnconnected=off
  wires:
  Triggered Subsystem/3(Out3) -> error3/1
  Sum/1 -> Compare To Zero/1
  Compare To Zero/1 -> Logical Operator/2
  Triggered Subsystem/2(Out2) -> error2/1
  Compare To Zero1/1 -> Logical Operator/1
  Logical Operator/1 -> Triggered Subsystem/Trigger, error triger/1
  Triggered Subsystem/1(Out1) -> error1/1, Memory/1
  Memory/1 -> Sum/2
  Error info/1 -> Sum/1, Triggered Subsystem/1(In1), Compare To Zero1/1

== system VCM_main/Error display Box/Error Info/error memory MC3 ==
  Error info : Inport
  Compare To Zero : simulink/Logic and Bit Operations/Compare To Zero  relop=~=  OutDataTypeStr=boolean
  Compare To Zero1 : simulink/Logic and Bit Operations/Compare To Zero  relop=~=  OutDataTypeStr=boolean
  Logical Operator : Logic  AllPortsSameDT=off  OutDataTypeStr=boolean
  Memory : Memory
  Sum : Sum  Inputs=|+-
  Triggered Subsystem : Subsystem  TreatAsAtomicUnit=on
  error1 : Outport  VectorParamsAs1DForOutWhenUnconnected=off
  error2 : Outport  Port=2  VectorParamsAs1DForOutWhenUnconnected=off
  error3 : Outport  Port=3  VectorParamsAs1DForOutWhenUnconnected=off
  error triger : Outport  Port=4  VectorParamsAs1DForOutWhenUnconnected=off
  wires:
  Triggered Subsystem/3(Out3) -> error3/1
  Sum/1 -> Compare To Zero/1
  Compare To Zero/1 -> Logical Operator/2
  Triggered Subsystem/2(Out2) -> error2/1
  Compare To Zero1/1 -> Logical Operator/1
  Logical Operator/1 -> Triggered Subsystem/Trigger, error triger/1
  Triggered Subsystem/1(Out1) -> error1/1, Memory/1
  Memory/1 -> Sum/2
  Error info/1 -> Sum/1, Triggered Subsystem/1(In1), Compare To Zero1/1

== system VCM_main/Error display Box/Error Info/error memory MC4 ==
  Error info : Inport
  Compare To Zero : simulink/Logic and Bit Operations/Compare To Zero  relop=~=  OutDataTypeStr=boolean
  Compare To Zero1 : simulink/Logic and Bit Operations/Compare To Zero  relop=~=  OutDataTypeStr=boolean
  Logical Operator : Logic  AllPortsSameDT=off  OutDataTypeStr=boolean
  Memory : Memory
  Sum : Sum  Inputs=|+-
  Triggered Subsystem : Subsystem  TreatAsAtomicUnit=on
  error1 : Outport  VectorParamsAs1DForOutWhenUnconnected=off
  error2 : Outport  Port=2  VectorParamsAs1DForOutWhenUnconnected=off
  error3 : Outport  Port=3  VectorParamsAs1DForOutWhenUnconnected=off
  error triger : Outport  Port=4  VectorParamsAs1DForOutWhenUnconnected=off
  wires:
  Triggered Subsystem/3(Out3) -> error3/1
  Sum/1 -> Compare To Zero/1
  Compare To Zero/1 -> Logical Operator/2
  Triggered Subsystem/2(Out2) -> error2/1
  Compare To Zero1/1 -> Logical Operator/1
  Logical Operator/1 -> Triggered Subsystem/Trigger, error triger/1
  Triggered Subsystem/1(Out1) -> error1/1, Memory/1
  Memory/1 -> Sum/2
  Error info/1 -> Sum/1, Triggered Subsystem/1(In1), Compare To Zero1/1

== system VCM_main/Error display Box/Error Info1/error memory MC1 ==
  Error info : Inport
  Error triger : Inport  Port=2
  Triggered Subsystem : Subsystem  TreatAsAtomicUnit=on
  error1 : Outport  VectorParamsAs1DForOutWhenUnconnected=off
  error2 : Outport  Port=2  VectorParamsAs1DForOutWhenUnconnected=off
  error3 : Outport  Port=3  VectorParamsAs1DForOutWhenUnconnected=off
  wires:
  Triggered Subsystem/3(Out3) -> error3/1
  Error triger/1 -> Triggered Subsystem/Trigger
  Triggered Subsystem/2(Out2) -> error2/1
  Triggered Subsystem/1(Out1) -> error1/1
  Error info/1 -> Triggered Subsystem/1(In1)

== system VCM_main/Error display Box/Error Info1/error memory MC2 ==
  Error info : Inport
  Error triger : Inport  Port=2
  Triggered Subsystem : Subsystem  TreatAsAtomicUnit=on
  error1 : Outport  VectorParamsAs1DForOutWhenUnconnected=off
  error2 : Outport  Port=2  VectorParamsAs1DForOutWhenUnconnected=off
  error3 : Outport  Port=3  VectorParamsAs1DForOutWhenUnconnected=off
  wires:
  Triggered Subsystem/3(Out3) -> error3/1
  Error triger/1 -> Triggered Subsystem/Trigger
  Triggered Subsystem/2(Out2) -> error2/1
  Triggered Subsystem/1(Out1) -> error1/1
  Error info/1 -> Triggered Subsystem/1(In1)

== system VCM_main/Error display Box/Error Info1/error memory MC3 ==
  Error info : Inport
  Error triger : Inport  Port=2
  Triggered Subsystem : Subsystem  TreatAsAtomicUnit=on
  error1 : Outport  VectorParamsAs1DForOutWhenUnconnected=off
  error2 : Outport  Port=2  VectorParamsAs1DForOutWhenUnconnected=off
  error3 : Outport  Port=3  VectorParamsAs1DForOutWhenUnconnected=off
  wires:
  Triggered Subsystem/3(Out3) -> error3/1
  Error triger/1 -> Triggered Subsystem/Trigger
  Triggered Subsystem/2(Out2) -> error2/1
  Triggered Subsystem/1(Out1) -> error1/1
  Error info/1 -> Triggered Subsystem/1(In1)

== system VCM_main/Error display Box/Error Info1/error memory MC4 ==
  Error info : Inport
  Error triger : Inport  Port=2
  Triggered Subsystem : Subsystem  TreatAsAtomicUnit=on
  error1 : Outport  VectorParamsAs1DForOutWhenUnconnected=off
  error2 : Outport  Port=2  VectorParamsAs1DForOutWhenUnconnected=off
  error3 : Outport  Port=3  VectorParamsAs1DForOutWhenUnconnected=off
  wires:
  Triggered Subsystem/3(Out3) -> error3/1
  Error triger/1 -> Triggered Subsystem/Trigger
  Triggered Subsystem/2(Out2) -> error2/1
  Triggered Subsystem/1(Out1) -> error1/1
  Error info/1 -> Triggered Subsystem/1(In1)

== system VCM_main/Error display Box/Error Info2/error memory MC1 ==
  Error info : Inport
  Error triger : Inport  Port=2
  Triggered Subsystem : Subsystem  TreatAsAtomicUnit=on
  error1 : Outport  VectorParamsAs1DForOutWhenUnconnected=off
  error2 : Outport  Port=2  VectorParamsAs1DForOutWhenUnconnected=off
  error3 : Outport  Port=3  VectorParamsAs1DForOutWhenUnconnected=off
  wires:
  Triggered Subsystem/3(Out3) -> error3/1
  Error triger/1 -> Triggered Subsystem/Trigger
  Triggered Subsystem/2(Out2) -> error2/1
  Triggered Subsystem/1(Out1) -> error1/1
  Error info/1 -> Triggered Subsystem/1(In1)

== system VCM_main/Error display Box/Error Info2/error memory MC2 ==
  Error info : Inport
  Error triger : Inport  Port=2
  Triggered Subsystem : Subsystem  TreatAsAtomicUnit=on
  error1 : Outport  VectorParamsAs1DForOutWhenUnconnected=off
  error2 : Outport  Port=2  VectorParamsAs1DForOutWhenUnconnected=off
  error3 : Outport  Port=3  VectorParamsAs1DForOutWhenUnconnected=off
  wires:
  Triggered Subsystem/3(Out3) -> error3/1
  Error triger/1 -> Triggered Subsystem/Trigger
  Triggered Subsystem/2(Out2) -> error2/1
  Triggered Subsystem/1(Out1) -> error1/1
  Error info/1 -> Triggered Subsystem/1(In1)

== system VCM_main/Error display Box/Error Info2/error memory MC3 ==
  Error info : Inport
  Error triger : Inport  Port=2
  Triggered Subsystem : Subsystem  TreatAsAtomicUnit=on
  error1 : Outport  VectorParamsAs1DForOutWhenUnconnected=off
  error2 : Outport  Port=2  VectorParamsAs1DForOutWhenUnconnected=off
  error3 : Outport  Port=3  VectorParamsAs1DForOutWhenUnconnected=off
  wires:
  Triggered Subsystem/3(Out3) -> error3/1
  Error triger/1 -> Triggered Subsystem/Trigger
  Triggered Subsystem/2(Out2) -> error2/1
  Triggered Subsystem/1(Out1) -> error1/1
  Error info/1 -> Triggered Subsystem/1(In1)

== system VCM_main/Error display Box/Error Info2/error memory MC4 ==
  Error info : Inport
  Error triger : Inport  Port=2
  Triggered Subsystem : Subsystem  TreatAsAtomicUnit=on
  error1 : Outport  VectorParamsAs1DForOutWhenUnconnected=off
  error2 : Outport  Port=2  VectorParamsAs1DForOutWhenUnconnected=off
  error3 : Outport  Port=3  VectorParamsAs1DForOutWhenUnconnected=off
  wires:
  Triggered Subsystem/3(Out3) -> error3/1
  Error triger/1 -> Triggered Subsystem/Trigger
  Triggered Subsystem/2(Out2) -> error2/1
  Triggered Subsystem/1(Out1) -> error1/1
  Error info/1 -> Triggered Subsystem/1(In1)

== system VCM_main/Error display Box/Error Info3/error memory MC1 ==
  Error info : Inport
  Error triger : Inport  Port=2
  Triggered Subsystem : Subsystem  TreatAsAtomicUnit=on
  error1 : Outport  VectorParamsAs1DForOutWhenUnconnected=off
  error2 : Outport  Port=2  VectorParamsAs1DForOutWhenUnconnected=off
  error3 : Outport  Port=3  VectorParamsAs1DForOutWhenUnconnected=off
  wires:
  Triggered Subsystem/3(Out3) -> error3/1
  Error triger/1 -> Triggered Subsystem/Trigger
  Triggered Subsystem/2(Out2) -> error2/1
  Triggered Subsystem/1(Out1) -> error1/1
  Error info/1 -> Triggered Subsystem/1(In1)

== system VCM_main/Error display Box/Error Info3/error memory MC2 ==
  Error info : Inport
  Error triger : Inport  Port=2
  Triggered Subsystem : Subsystem  TreatAsAtomicUnit=on
  error1 : Outport  VectorParamsAs1DForOutWhenUnconnected=off
  error2 : Outport  Port=2  VectorParamsAs1DForOutWhenUnconnected=off
  error3 : Outport  Port=3  VectorParamsAs1DForOutWhenUnconnected=off
  wires:
  Triggered Subsystem/3(Out3) -> error3/1
  Error triger/1 -> Triggered Subsystem/Trigger
  Triggered Subsystem/2(Out2) -> error2/1
  Triggered Subsystem/1(Out1) -> error1/1
  Error info/1 -> Triggered Subsystem/1(In1)

== system VCM_main/Error display Box/Error Info3/error memory MC3 ==
  Error info : Inport
  Error triger : Inport  Port=2
  Triggered Subsystem : Subsystem  TreatAsAtomicUnit=on
  error1 : Outport  VectorParamsAs1DForOutWhenUnconnected=off
  error2 : Outport  Port=2  VectorParamsAs1DForOutWhenUnconnected=off
  error3 : Outport  Port=3  VectorParamsAs1DForOutWhenUnconnected=off
  wires:
  Triggered Subsystem/3(Out3) -> error3/1
  Error triger/1 -> Triggered Subsystem/Trigger
  Triggered Subsystem/2(Out2) -> error2/1
  Triggered Subsystem/1(Out1) -> error1/1
  Error info/1 -> Triggered Subsystem/1(In1)
